simulink model "Quadrotor"  (Simulink 7.7)
settings: Solver=ode23tb  StartTime=0.0  StopTime=140  MaxStep=1e-3  RelTol=1e-3
values from neighbouring files (symbols this model uses):
  b = 54.2e-6    (= 5.42e-05)    [ParamQuadrotor.m]
  d = 1.1e-6    (= 1.1e-06)    [ParamQuadrotor.m]
  g = 9.81    [ParamQuadrotor.m]
  h = 1e-3    (= 0.001)    [ParamQuadrotor.m]
  Ixx = 8.1e-3    (= 0.0081)    [ParamQuadrotor.m]
  Iyy = 8.1e-3    (= 0.0081)    [ParamQuadrotor.m]
  Izz = 14.2e-3    (= 0.0142)    [ParamQuadrotor.m]
  Jtp = 104e-6    (= 0.000104)    [ParamQuadrotor.m]
  Kd_angle = 10*2    (= 20)    [ParamQuadrotor.m]
  Kd_motor = 0    [ParamQuadrotor.m]
  Kd_position = 10    [ParamQuadrotor.m]
  Ke = 6.3e-3    (= 0.0063)    [ParamQuadrotor.m]
  Ki_angle = 0    [ParamQuadrotor.m]
  Ki_motor = 10    [ParamQuadrotor.m]
  Ki_position = 0    [ParamQuadrotor.m]
  Km = 6.3e-3    (= 0.0063)    [ParamQuadrotor.m]
  Kp_angle = 5*2    (= 10)    [ParamQuadrotor.m]
  Kp_motor = 1    [ParamQuadrotor.m]
  Kp_position = 5    [ParamQuadrotor.m]
  l = 0.24    [ParamQuadrotor.m]
  m = 1    [ParamQuadrotor.m]
  n = 0.9    [ParamQuadrotor.m]
  N = 5.6    [ParamQuadrotor.m]
  R = 0.6    [ParamQuadrotor.m]
undefined symbols (not defined in the file or in its folder): Newton, Raphson
libraries: simulink x10
settings Model: Creator=hts  LastModifiedBy=Tai-Sik
settings SFSimCC: SimParseCustomCode=off

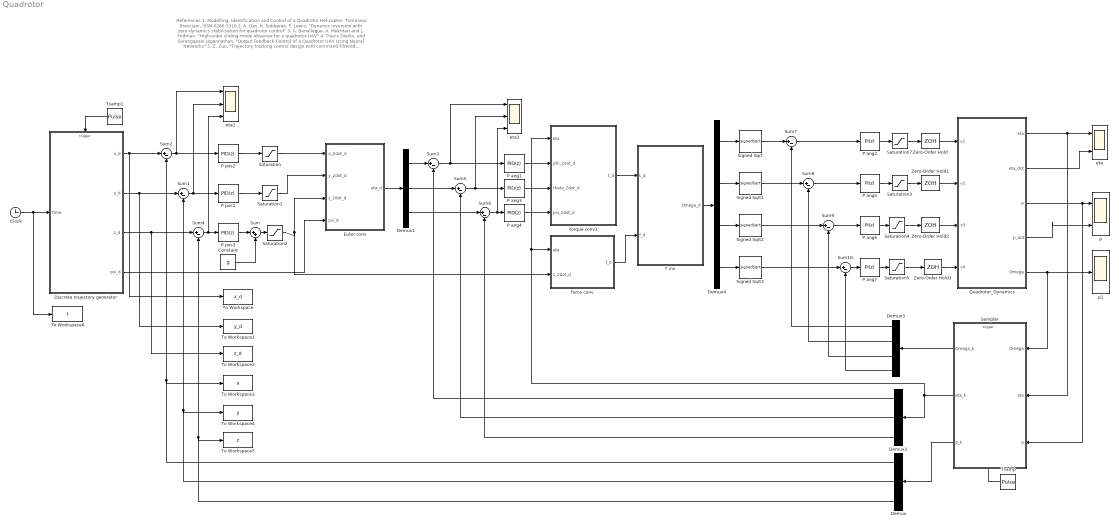
== system Quadrotor ==
  note: References
      | 1. Modelling, Identification and Control
      | of a Quadrotor Helicopter, Tommaso Bresciani, ISSN 0280-5316
      | 2. A. Das, K. Subbarao, F. Lewis, "Dynamic inversion with zero-dynamics
      | stabilisation for quadrotor control"
      | 3. A. Benallegue, A. Mokhtari and L. Fridman, "High-order sliding-mode observer for a quadrotor UAV"
      | 4. Travis Dierks, and Sarangapani Jagannathan, "Output Feedback Control of a Quadrotor UAV Using Neural Networks"
      | 5. Z. Zuo, "Trajectory tracking control design with command-filtered compensation for a quadrotor"
  Clock : Clock
      settings: Decimation=10
  Constant : Constant  Value=g
  Demux : Demux  Outputs=3
  Demux1 : Demux  Outputs=3
  Demux2 : Demux  Outputs=3
  Demux3 : Demux
  Demux4 : Demux
  Discrete trajectory generator : Subsystem  TreatAsAtomicUnit=on
  Euler conv : Stateflow chart  TreatAsAtomicUnit=on
  P ang1 : simulink/Continuous/PID Controller  SystemSampleTime=-1  Controller=PID  TimeDomain=Discrete-time  SampleTime=h  IntegratorMethod=Trapezoidal  FilterMethod=Trapezoidal  Form=Parallel  P=Kp_angle  I=Ki_angle  D=Kd_angle  N=100  InitialConditionSource=internal  InitialConditionForIntegrator=0  InitialConditionForFilter=0  ExternalReset=none  LimitOutput=off  UpperSaturationLimit=inf  LowerSaturationLimit=-inf  LinearizeAsGain=off  AntiWindupMode=none  Kb=1  TrackingMode=off  Kt=1  PParamMin=[]  PParamMax=[]  IParamMin=[]  IParamMax=[]  DParamMin=[]  DParamMax=[]  NParamMin=[]  NParamMax=[]  KbParamMin=[]  KbParamMax=[]  KtParamMin=[]  KtParamMax=[]  POutMin=[]  POutMax=[]  IOutMin=[]  IOutMax=[]  DOutMin=[]  DOutMax=[]  NOutMin=[]  NOutMax=[]  KbOutMin=[]  KbOutMax=[]  KtOutMin=[]  KtOutMax=[]  IntegratorOutMin=[]  IntegratorOutMax=[]  FilterOutMin=[]  FilterOutMax=[]  SumOutMin=[]  SumOutMax=[]  SumI1OutMin=[]  SumI1OutMax=[]  SumI2OutMin=[]  SumI2OutMax=[]  SumI3OutMin=[]  SumI3OutMax=[]  SumDOutMin=[]  SumDOutMax=[]  SaturationOutMin=[]  SaturationOutMax=[]  IntegratorContinuousStateAttributes=''  IntegratorStateMustResolveToSignalObject=off  IntegratorRTWStateStorageClass=Auto  FilterContinuousStateAttributes=''  FilterStateMustResolveToSignalObject=off  FilterRTWStateStorageClass=Auto
  P ang{2,5..7} (4 alike) : simulink/Continuous/PID Controller  SystemSampleTime=-1  Controller=PI  TimeDomain=Discrete-time  SampleTime=h  IntegratorMethod=Trapezoidal  FilterMethod=Trapezoidal  Form=Parallel  P=Kp_motor  I=Ki_motor  D=Kd_motor  N=100  InitialConditionSource=internal  InitialConditionForIntegrator=0  InitialConditionForFilter=0  ExternalReset=none  LimitOutput=off  UpperSaturationLimit=inf  LowerSaturationLimit=-inf  LinearizeAsGain=off  AntiWindupMode=none  Kb=1  TrackingMode=off  Kt=1  PParamMin=[]  PParamMax=[]  IParamMin=[]  IParamMax=[]  DParamMin=[]  DParamMax=[]  NParamMin=[]  NParamMax=[]  KbParamMin=[]  KbParamMax=[]  KtParamMin=[]  KtParamMax=[]  POutMin=[]  POutMax=[]  IOutMin=[]  IOutMax=[]  DOutMin=[]  DOutMax=[]  NOutMin=[]  NOutMax=[]  KbOutMin=[]  KbOutMax=[]  KtOutMin=[]  KtOutMax=[]  IntegratorOutMin=[]  IntegratorOutMax=[]  FilterOutMin=[]  FilterOutMax=[]  SumOutMin=[]  SumOutMax=[]  SumI1OutMin=[]  SumI1OutMax=[]  SumI2OutMin=[]  SumI2OutMax=[]  SumI3OutMin=[]  SumI3OutMax=[]  SumDOutMin=[]  SumDOutMax=[]  SaturationOutMin=[]  SaturationOutMax=[]  IntegratorContinuousStateAttributes=''  IntegratorStateMustResolveToSignalObject=off  IntegratorRTWStateStorageClass=Auto  FilterContinuousStateAttributes=''  FilterStateMustResolveToSignalObject=off  FilterRTWStateStorageClass=Auto
  P ang3 : simulink/Continuous/PID Controller  SystemSampleTime=-1  Controller=PID  TimeDomain=Discrete-time  SampleTime=h  IntegratorMethod=Trapezoidal  FilterMethod=Trapezoidal  Form=Parallel  P=Kp_angle  I=Ki_angle  D=Kd_angle  N=100  InitialConditionSource=internal  InitialConditionForIntegrator=0  InitialConditionForFilter=0  ExternalReset=none  LimitOutput=off  UpperSaturationLimit=inf  LowerSaturationLimit=-inf  LinearizeAsGain=off  AntiWindupMode=none  Kb=1  TrackingMode=off  Kt=1  PParamMin=[]  PParamMax=[]  IParamMin=[]  IParamMax=[]  DParamMin=[]  DParamMax=[]  NParamMin=[]  NParamMax=[]  KbParamMin=[]  KbParamMax=[]  KtParamMin=[]  KtParamMax=[]  POutMin=[]  POutMax=[]  IOutMin=[]  IOutMax=[]  DOutMin=[]  DOutMax=[]  NOutMin=[]  NOutMax=[]  KbOutMin=[]  KbOutMax=[]  KtOutMin=[]  KtOutMax=[]  IntegratorOutMin=[]  IntegratorOutMax=[]  FilterOutMin=[]  FilterOutMax=[]  SumOutMin=[]  SumOutMax=[]  SumI1OutMin=[]  SumI1OutMax=[]  SumI2OutMin=[]  SumI2OutMax=[]  SumI3OutMin=[]  SumI3OutMax=[]  SumDOutMin=[]  SumDOutMax=[]  SaturationOutMin=[]  SaturationOutMax=[]  IntegratorContinuousStateAttributes=''  IntegratorStateMustResolveToSignalObject=off  IntegratorRTWStateStorageClass=Auto  FilterContinuousStateAttributes=''  FilterStateMustResolveToSignalObject=off  FilterRTWStateStorageClass=Auto
  P ang4 : simulink/Continuous/PID Controller  SystemSampleTime=-1  Controller=PID  TimeDomain=Discrete-time  SampleTime=h  IntegratorMethod=Trapezoidal  FilterMethod=Trapezoidal  Form=Parallel  P=Kp_angle  I=Ki_angle  D=Kd_angle  N=100  InitialConditionSource=internal  InitialConditionForIntegrator=0  InitialConditionForFilter=0  ExternalReset=none  LimitOutput=off  UpperSaturationLimit=inf  LowerSaturationLimit=-inf  LinearizeAsGain=off  AntiWindupMode=none  Kb=1  TrackingMode=off  Kt=1  PParamMin=[]  PParamMax=[]  IParamMin=[]  IParamMax=[]  DParamMin=[]  DParamMax=[]  NParamMin=[]  NParamMax=[]  KbParamMin=[]  KbParamMax=[]  KtParamMin=[]  KtParamMax=[]  POutMin=[]  POutMax=[]  IOutMin=[]  IOutMax=[]  DOutMin=[]  DOutMax=[]  NOutMin=[]  NOutMax=[]  KbOutMin=[]  KbOutMax=[]  KtOutMin=[]  KtOutMax=[]  IntegratorOutMin=[]  IntegratorOutMax=[]  FilterOutMin=[]  FilterOutMax=[]  SumOutMin=[]  SumOutMax=[]  SumI1OutMin=[]  SumI1OutMax=[]  SumI2OutMin=[]  SumI2OutMax=[]  SumI3OutMin=[]  SumI3OutMax=[]  SumDOutMin=[]  SumDOutMax=[]  SaturationOutMin=[]  SaturationOutMax=[]  IntegratorContinuousStateAttributes=''  IntegratorStateMustResolveToSignalObject=off  IntegratorRTWStateStorageClass=Auto  FilterContinuousStateAttributes=''  FilterStateMustResolveToSignalObject=off  FilterRTWStateStorageClass=Auto
  P pos1 : simulink/Continuous/PID Controller  SystemSampleTime=-1  Controller=PID  TimeDomain=Discrete-time  SampleTime=h  IntegratorMethod=Trapezoidal  FilterMethod=Trapezoidal  Form=Parallel  P=Kp_position  I=Ki_position  D=Kd_position  N=100  InitialConditionSource=internal  InitialConditionForIntegrator=0  InitialConditionForFilter=0  ExternalReset=none  LimitOutput=off  UpperSaturationLimit=5  LowerSaturationLimit=-10  LinearizeAsGain=off  AntiWindupMode=none  Kb=1  TrackingMode=off  Kt=1  PParamMin=[]  PParamMax=[]  IParamMin=[]  IParamMax=[]  DParamMin=[]  DParamMax=[]  NParamMin=[]  NParamMax=[]  KbParamMin=[]  KbParamMax=[]  KtParamMin=[]  KtParamMax=[]  POutMin=[]  POutMax=[]  IOutMin=[]  IOutMax=[]  DOutMin=[]  DOutMax=[]  NOutMin=[]  NOutMax=[]  KbOutMin=[]  KbOutMax=[]  KtOutMin=[]  KtOutMax=[]  IntegratorOutMin=[]  IntegratorOutMax=[]  FilterOutMin=[]  FilterOutMax=[]  SumOutMin=[]  SumOutMax=[]  SumI1OutMin=[]  SumI1OutMax=[]  SumI2OutMin=[]  SumI2OutMax=[]  SumI3OutMin=[]  SumI3OutMax=[]  SumDOutMin=[]  SumDOutMax=[]  SaturationOutMin=[]  SaturationOutMax=[]  IntegratorContinuousStateAttributes=''  IntegratorStateMustResolveToSignalObject=off  IntegratorRTWStateStorageClass=Auto  FilterContinuousStateAttributes=''  FilterStateMustResolveToSignalObject=off  FilterRTWStateStorageClass=Auto
  P pos2 : simulink/Continuous/PID Controller  SystemSampleTime=-1  Controller=PID  TimeDomain=Discrete-time  SampleTime=h  IntegratorMethod=Trapezoidal  FilterMethod=Trapezoidal  Form=Parallel  P=Kp_position  I=Ki_position  D=Kd_position  N=100  InitialConditionSource=internal  InitialConditionForIntegrator=0  InitialConditionForFilter=0  ExternalReset=none  LimitOutput=off  UpperSaturationLimit=5  LowerSaturationLimit=-10  LinearizeAsGain=off  AntiWindupMode=none  Kb=1  TrackingMode=off  Kt=1  PParamMin=[]  PParamMax=[]  IParamMin=[]  IParamMax=[]  DParamMin=[]  DParamMax=[]  NParamMin=[]  NParamMax=[]  KbParamMin=[]  KbParamMax=[]  KtParamMin=[]  KtParamMax=[]  POutMin=[]  POutMax=[]  IOutMin=[]  IOutMax=[]  DOutMin=[]  DOutMax=[]  NOutMin=[]  NOutMax=[]  KbOutMin=[]  KbOutMax=[]  KtOutMin=[]  KtOutMax=[]  IntegratorOutMin=[]  IntegratorOutMax=[]  FilterOutMin=[]  FilterOutMax=[]  SumOutMin=[]  SumOutMax=[]  SumI1OutMin=[]  SumI1OutMax=[]  SumI2OutMin=[]  SumI2OutMax=[]  SumI3OutMin=[]  SumI3OutMax=[]  SumDOutMin=[]  SumDOutMax=[]  SaturationOutMin=[]  SaturationOutMax=[]  IntegratorContinuousStateAttributes=''  IntegratorStateMustResolveToSignalObject=off  IntegratorRTWStateStorageClass=Auto  FilterContinuousStateAttributes=''  FilterStateMustResolveToSignalObject=off  FilterRTWStateStorageClass=Auto
  P pos3 : simulink/Continuous/PID Controller  SystemSampleTime=-1  Controller=PID  TimeDomain=Discrete-time  SampleTime=h  IntegratorMethod=Trapezoidal  FilterMethod=Trapezoidal  Form=Parallel  P=Kp_position  I=Ki_position  D=Kd_position  N=100  InitialConditionSource=internal  InitialConditionForIntegrator=0  InitialConditionForFilter=0  ExternalReset=none  LimitOutput=off  UpperSaturationLimit=5  LowerSaturationLimit=-10  LinearizeAsGain=off  AntiWindupMode=none  Kb=1  TrackingMode=off  Kt=1  PParamMin=[]  PParamMax=[]  IParamMin=[]  IParamMax=[]  DParamMin=[]  DParamMax=[]  NParamMin=[]  NParamMax=[]  KbParamMin=[]  KbParamMax=[]  KtParamMin=[]  KtParamMax=[]  POutMin=[]  POutMax=[]  IOutMin=[]  IOutMax=[]  DOutMin=[]  DOutMax=[]  NOutMin=[]  NOutMax=[]  KbOutMin=[]  KbOutMax=[]  KtOutMin=[]  KtOutMax=[]  IntegratorOutMin=[]  IntegratorOutMax=[]  FilterOutMin=[]  FilterOutMax=[]  SumOutMin=[]  SumOutMax=[]  SumI1OutMin=[]  SumI1OutMax=[]  SumI2OutMin=[]  SumI2OutMax=[]  SumI3OutMin=[]  SumI3OutMax=[]  SumDOutMin=[]  SumDOutMax=[]  SaturationOutMin=[]  SaturationOutMax=[]  IntegratorContinuousStateAttributes=''  IntegratorStateMustResolveToSignalObject=off  IntegratorRTWStateStorageClass=Auto  FilterContinuousStateAttributes=''  FilterStateMustResolveToSignalObject=off  FilterRTWStateStorageClass=Auto
  Quadrotor_Dynamics : Subsystem
  Sampler : Subsystem  TreatAsAtomicUnit=on
  Saturation : Saturate  UpperLimit=3*g  LowerLimit=-3*g
  Saturation1 : Saturate  UpperLimit=3*g  LowerLimit=-3*g
  Saturation2 : Saturate  UpperLimit=3*g  LowerLimit=-3*g
  Saturation{3..5,7} (4 alike) : Saturate  UpperLimit=100  LowerLimit=-100
  Signed Sqrt{,1..3} (4 alike) : Sqrt  Operator=signedSqrt  AlgorithmType=Newton-Raphson  SaturateOnIntegerOverflow=on
  Sum : Sum  Inputs=|++
  Sum{1..10} (10 alike) : Sum  Inputs=|+-
  T inv : Stateflow chart  TreatAsAtomicUnit=on
  To Workspace : ToWorkspace  VariableName=x_d  SampleTime=h*10  SaveFormat=Array
  To Workspace1 : ToWorkspace  VariableName=y_d  SampleTime=h*10  SaveFormat=Array
  To Workspace2 : ToWorkspace  VariableName=z_d  SampleTime=h*10  SaveFormat=Array
  To Workspace3 : ToWorkspace  VariableName=x  SampleTime=h*10  SaveFormat=Array
  To Workspace4 : ToWorkspace  VariableName=y  SampleTime=h*10  SaveFormat=Array
  To Workspace5 : ToWorkspace  VariableName=z  SampleTime=h*10  SaveFormat=Array
  To Workspace6 : ToWorkspace  VariableName=t  SampleTime=h*10  SaveFormat=Array
  Tsamp : DiscretePulseGenerator  PulseType=Time based  Period=h  PulseWidth=50
  Tsamp1 : DiscretePulseGenerator  PulseType=Time based  Period=h  PulseWidth=50
  Zero-Order Hold{,1..3} (4 alike) : ZeroOrderHold  SampleTime=h
  eta : Scope  NumInputPorts=2
      settings: TimeRange=20  YMin=-0.1~-1.75  YMax=0.55~1
  eta1 : Scope  NumInputPorts=3
      settings: TimeRange=20  YMin=-0.4~0.05~0.14  YMax=0.4~0.4~0.18  SaveName=ScopeData5
  eta2 : Scope  NumInputPorts=3
      settings: TimeRange=20  YMin=-0.275~-0.275~-0.03  YMax=0.1~0.1~0.06  SaveName=ScopeData6
  force conv : Stateflow chart  TreatAsAtomicUnit=on
  p : Scope  NumInputPorts=2
      settings: TimeRange=80  YMin=0~0  YMax=20~2.75
  p1 : Scope
      settings: TimeRange=0.7000000000000001  YMin=213.268  YMax=213.31  SaveName=ScopeData4
  torque conv1 : Stateflow chart  TreatAsAtomicUnit=on
  wires:
  Quadrotor_Dynamics/1(eta) -> eta/1, Sampler/2(eta)
  Quadrotor_Dynamics/3(p) -> p/1, Sampler/3(p)
  Sum4/1 -> P pos3/1, eta1/3
  Discrete trajectory generator/3(z_d) -> Sum4/1, To Workspace2/1
  P pos3/1 -> Sum/1
  Sum/1 -> Saturation2/1
  Sum1/1 -> P pos1/1, eta1/2
  Discrete trajectory generator/2(y_d) -> Sum1/1, To Workspace1/1
  Sum2/1 -> P pos2/1, eta1/1
  Discrete trajectory generator/1(x_d) -> Sum2/1, To Workspace/1
  P pos2/1 -> Saturation/1
  P pos1/1 -> Saturation1/1
  Sum3/1 -> P ang1/1, eta2/1
  Sum5/1 -> P ang3/1, eta2/2
  Sum6/1 -> P ang4/1, eta2/3
  Demux2/1 -> Sum3/2
  Demux2/2 -> Sum5/2
  Demux2/3 -> Sum6/2
  P ang1/1 -> torque conv1/2(phi_2dot_d)
  P ang3/1 -> torque conv1/3(theta_2dot_d)
  P ang4/1 -> torque conv1/4(psi_2dot_d)
  Saturation2/1 -> force conv/2(z_2dot_d), Euler conv/3(z_2dot_d)
  Constant/1 -> Sum/2
  Demux1/1 -> Sum3/1
  Demux1/2 -> Sum5/1
  Saturation/1 -> Euler conv/1(x_2dot_d)
  Saturation1/1 -> Euler conv/2(y_2dot_d)
  Euler conv/1(eta_d) -> Demux1/1
  Demux1/3 -> Sum6/1
  Demux/1 -> Sum2/2, To Workspace3/1
  Demux/2 -> Sum1/2, To Workspace4/1
  Demux/3 -> Sum4/2, To Workspace5/1
  Tsamp/1 -> Sampler/Trigger
  Sampler/1(Omega_k) -> Demux3/1
  Sampler/3(p_k) -> Demux/1
  Quadrotor_Dynamics/5(Omega) -> Sampler/1(Omega), p1/1
  torque conv1/1(t_d) -> T inv/1(t_d)
  force conv/1(f_d) -> T inv/2(f_d)
  Sampler/2(eta_k) -> Demux2/1, force conv/1(eta), torque conv1/1(eta)
  Demux4/1 -> Signed Sqrt/1
  Sum7/1 -> P ang2/1
  Demux3/1 -> Sum7/2
  Demux4/2 -> Signed Sqrt1/1
  Demux4/4 -> Signed Sqrt3/1
  Sum8/1 -> P ang5/1
  Demux3/2 -> Sum8/2
  Demux3/3 -> Sum9/2
  Sum9/1 -> P ang6/1
  Sum10/1 -> P ang7/1
  Demux3/4 -> Sum10/2
  P ang2/1 -> Saturation7/1
  P ang5/1 -> Saturation3/1
  P ang6/1 -> Saturation4/1
  P ang7/1 -> Saturation5/1
  Demux4/3 -> Signed Sqrt2/1
  Zero-Order Hold/1 -> Quadrotor_Dynamics/1(v1)
  Zero-Order Hold1/1 -> Quadrotor_Dynamics/2(v2)
  Zero-Order Hold2/1 -> Quadrotor_Dynamics/3(v3)
  Zero-Order Hold3/1 -> Quadrotor_Dynamics/4(v4)
  Saturation7/1 -> Zero-Order Hold/1
  Saturation3/1 -> Zero-Order Hold1/1
  Saturation4/1 -> Zero-Order Hold2/1
  Saturation5/1 -> Zero-Order Hold3/1
  T inv/1(Omega_d) -> Demux4/1
  Signed Sqrt/1 -> Sum7/1
  Signed Sqrt1/1 -> Sum8/1
  Signed Sqrt2/1 -> Sum9/1
  Signed Sqrt3/1 -> Sum10/1
  Discrete trajectory generator/4(psi_d) -> Euler conv/4(psi_d)
  Tsamp1/1 -> Discrete trajectory generator/Trigger
  Clock/1 -> Discrete trajectory generator/1(Time), To Workspace6/1
  Quadrotor_Dynamics/2(eta_dot) -> eta/2
  Quadrotor_Dynamics/4(p_dot) -> p/2

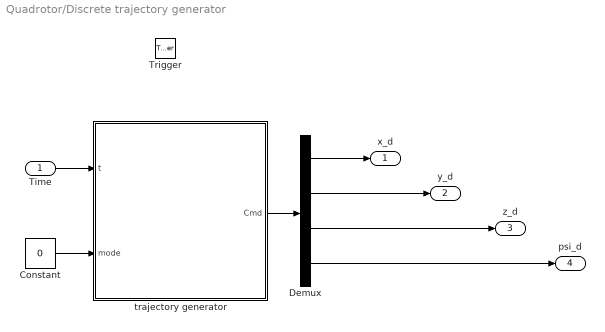
== system Quadrotor/Discrete trajectory generator ==
  Time : Inport
  Trigger : TriggerPort
  Constant : Constant  Value=0
  Demux : Demux
  trajectory generator : Stateflow chart  TreatAsAtomicUnit=on
  x_d : Outport
  y_d : Outport  Port=2
  z_d : Outport  Port=3
  psi_d : Outport  Port=4
  wires:
  Time/1 -> trajectory generator/1(t)
  trajectory generator/1(Cmd) -> Demux/1
  Demux/1 -> x_d/1
  Demux/2 -> y_d/1
  Demux/3 -> z_d/1
  Demux/4 -> psi_d/1
  Constant/1 -> trajectory generator/2(mode)

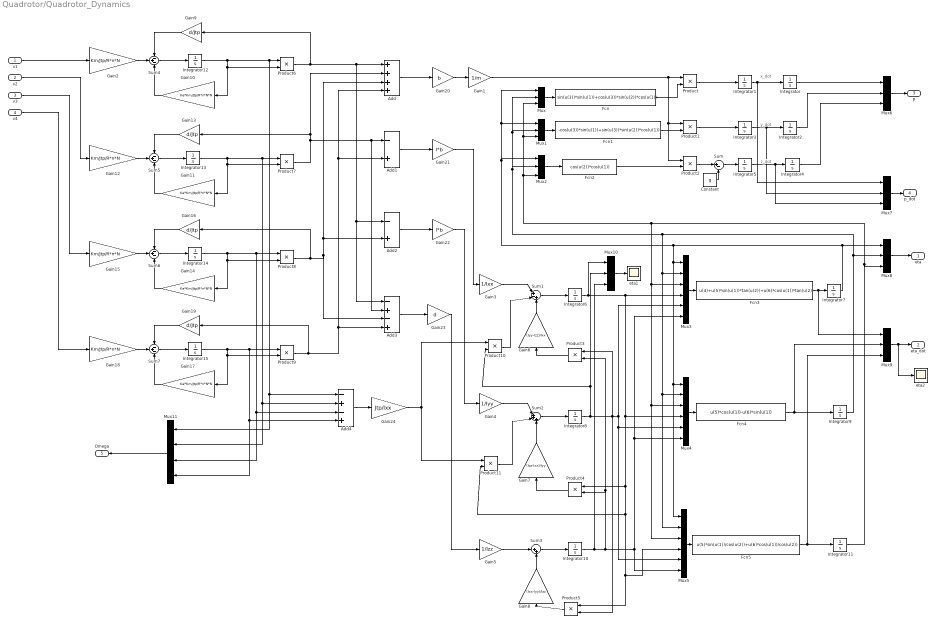
== system Quadrotor/Quadrotor_Dynamics ==
  note: x_dot
  note: y_dot
  note: z_dot
  v1 : Inport
  v2 : Inport  Port=2
  v3 : Inport  Port=3
  v4 : Inport  Port=4
  Add : Sum  Inputs=++++
  Add1 : Sum  Inputs=-+
  Add2 : Sum  Inputs=-+
  Add3 : Sum  Inputs=-+-+
  Add4 : Sum  Inputs=-+-+
  Constant : Constant  Value=g
  Fcn : Fcn  Expr=sin(u(3))*sin(u(1))+cos(u(3))*sin(u(2))*cos(u(1))
  Fcn1 : Fcn  Expr=-cos(u(3))*sin(u(1))+sin(u(3))*sin(u(2))*cos(u(1))
  Fcn2 : Fcn  Expr=cos(u(2))*cos(u(1))
  Fcn3 : Fcn  Expr=u(4)+u(5)*sin(u(1))*tan(u(2))+u(6)*cos(u(1))*tan(u(2))
  Fcn4 : Fcn  Expr=u(5)*cos(u(1))-u(6)*sin(u(1))
  Fcn5 : Fcn  Expr=u(5)*sin(u(1))/cos(u(2))+u(6)*cos(u(1))/cos(u(2))
  Gain1 : Gain  Gain=1/m
  Gain{10..11,14,17} (4 alike) : Gain  Gain=Ke*Km/Jtp/R*n*N*N
  Gain{2,12,15,18} (4 alike) : Gain  Gain=Km/Jtp/R*n*N
  Gain{9,13,16,19} (4 alike) : Gain  Gain=d/Jtp
  Gain20 : Gain  Gain=b
  Gain21 : Gain  Gain=l*b
  Gain22 : Gain  Gain=l*b
  Gain23 : Gain  Gain=d
  Gain24 : Gain  Gain=Jtp/Ixx
  Gain3 : Gain  Gain=1/Ixx
  Gain4 : Gain  Gain=1/Iyy
  Gain5 : Gain  Gain=1/Izz
  Gain6 : Gain  Gain=(Iyy-Izz)/Ixx
  Gain7 : Gain  Gain=(Izz-Ixx)/Iyy
  Gain8 : Gain  Gain=(Ixx-Iyy)/Izz
  Integrator{,1..15} (16 alike) : Integrator
  Mux{,1..2,6..10} (8 alike) : Mux  Inputs=3
  Mux11 : Mux
  Mux3 : Mux  Inputs=6
  Mux4 : Mux  Inputs=6
  Mux5 : Mux  Inputs=6
  Product{,1..11} (12 alike) : Product  RndMeth=Zero
  Sum : Sum  Inputs=|+-
  Sum1 : Sum  Inputs=|+-+
  Sum2 : Sum  Inputs=|+++
  Sum3 : Sum  Inputs=|++
  Sum{4..7} (4 alike) : Sum  Inputs=-+-
  eta1 : Scope
      settings: TimeRange=10  YMin=-0.00225  YMax=0.003  SaveName=ScopeData2
  eta2 : Scope
      settings: TimeRange=10  YMin=-0.0008  YMax=0.0008  SaveName=ScopeData3
  eta : Outport
  eta_dot : Outport  Port=2
  p : Outport  Port=3
  p_dot : Outport  Port=4
  Omega : Outport  Port=5
  wires:
  Integrator1/1 -> Integrator/1, Mux7/1
  Product/1 -> Integrator1/1
  Mux/1 -> Fcn/1
  Fcn/1 -> Product/2
  Integrator3/1 -> Integrator2/1, Mux7/2
  Product1/1 -> Integrator3/1
  Integrator5/1 -> Integrator4/1, Mux7/3
  Mux2/1 -> Fcn2/1
  Fcn2/1 -> Product2/2
  Product2/1 -> Sum/1
  Sum/1 -> Integrator5/1
  Constant/1 -> Sum/2
  Sum1/1 -> Integrator6/1
  Fcn3/1 -> Integrator7/1, Mux9/1
  Integrator7/1 -> Mux8/1, Mux3/1, Mux4/1, Mux5/1, Mux2/1, Mux1/1, Mux/1
  Mux3/1 -> Fcn3/1
  Integrator6/1 -> Mux3/4, Product4/1, Product5/1, Mux5/4, Product11/2, Mux4/4, Mux10/1
  Sum2/1 -> Integrator8/1
  Fcn4/1 -> Integrator9/1, Mux9/2
  Integrator9/1 -> Mux8/2, Mux3/2, Mux4/2, Mux5/2, Mux/2, Mux1/2, Mux2/2
  Mux4/1 -> Fcn4/1
  Integrator8/1 -> Product5/2, Product3/1, Mux3/5, Mux4/5, Mux5/5, Mux10/2, Product10/2
  Sum3/1 -> Integrator10/1
  Gain5/1 -> Sum3/1
  Fcn5/1 -> Integrator11/1, Mux9/3
  Integrator11/1 -> Mux8/3, Mux3/3, Mux4/3, Mux5/3, Mux/3, Mux1/3, Mux2/3
  Mux5/1 -> Fcn5/1
  Integrator10/1 -> Product3/2, Product4/2, Mux3/6, Mux4/6, Mux5/6, Mux10/3
  Product3/1 -> Gain6/1
  Product4/1 -> Gain7/1
  Product5/1 -> Gain8/1
  Gain8/1 -> Sum3/2
  Mux6/1 -> p/1
  Mux7/1 -> p_dot/1
  Mux8/1 -> eta/1
  Mux9/1 -> eta_dot/1, eta2/1
  Mux10/1 -> eta1/1
  Gain1/1 -> Product/1, Product2/1, Product1/1
  Gain2/1 -> Sum4/2
  Gain9/1 -> Sum4/1
  Gain10/1 -> Sum4/3
  Integrator12/1 -> Gain10/1, Product6/2, Product6/1, Add4/1, Mux11/1
  Product6/1 -> Gain9/1, Add/1, Add2/1, Add3/1
  Gain12/1 -> Sum5/2
  Gain13/1 -> Sum5/1
  Integrator13/1 -> Gain11/1, Product7/2, Product7/1, Add4/2, Mux11/2
  Product7/1 -> Gain13/1, Add/2, Add1/1, Add3/2
  Gain15/1 -> Sum6/2
  Gain16/1 -> Sum6/1
  Gain14/1 -> Sum6/3
  Integrator14/1 -> Gain14/1, Product8/2, Product8/1, Add4/3, Mux11/3
  Product8/1 -> Gain16/1, Add/3, Add2/2, Add3/3
  Gain18/1 -> Sum7/2
  Gain19/1 -> Sum7/1
  Gain17/1 -> Sum7/3
  Integrator15/1 -> Gain17/1, Product9/2, Product9/1, Add4/4, Mux11/4
  Product9/1 -> Gain19/1, Add/4, Add1/2, Add3/4
  Mux11/1 -> Omega/1
  Gain6/1 -> Sum1/3
  Gain3/1 -> Sum1/1
  Gain7/1 -> Sum2/3
  Gain4/1 -> Sum2/1
  Product10/1 -> Sum1/2
  Product11/1 -> Sum2/2
  v1/1 -> Gain2/1
  v2/1 -> Gain12/1
  v3/1 -> Gain15/1
  v4/1 -> Gain18/1
  Gain11/1 -> Sum5/3
  Gain20/1 -> Gain1/1
  Gain21/1 -> Gain3/1
  Gain22/1 -> Gain4/1
  Gain23/1 -> Gain5/1
  Sum6/1 -> Integrator14/1
  Sum7/1 -> Integrator15/1
  Sum4/1 -> Integrator12/1
  Sum5/1 -> Integrator13/1
  Add4/1 -> Gain24/1
  Add/1 -> Gain20/1
  Add1/1 -> Gain21/1
  Add2/1 -> Gain22/1
  Add3/1 -> Gain23/1
  Mux1/1 -> Fcn1/1
  Fcn1/1 -> Product1/2
  Integrator/1 -> Mux6/1
  Integrator2/1 -> Mux6/2
  Integrator4/1 -> Mux6/3
  Gain24/1 -> Product10/1, Product11/1

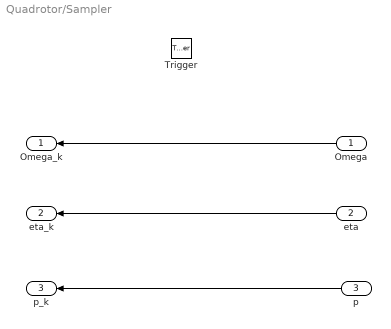
== system Quadrotor/Sampler ==
  Omega : Inport
  eta : Inport  Port=2
  p : Inport  Port=3
  Trigger : TriggerPort
  Omega_k : Outport
  eta_k : Outport  Port=2
  p_k : Outport  Port=3
  wires:
  Omega/1 -> Omega_k/1
  eta/1 -> eta_k/1
  p/1 -> p_k/1

== matlab function torque conv1 ==
  data: eta input double size=3; phi_2dot_d input double size=1; theta_2dot_d input double size=1; psi_2dot_d input double size=1; t_d output double size=3; I parameter double
function t_d = C(eta,phi_2dot_d,theta_2dot_d,psi_2dot_d,I)

tr_d = [phi_2dot_d;theta_2dot_d;psi_2dot_d];
sphi = sin(eta(1));
cphi = cos(eta(1));
stht = sin(eta(2));
ctht = cos(eta(2));
spsi = sin(eta(3));
cpsi = cos(eta(3));

C = [1   0     -stht;
     0   cphi  sphi*ctht;
     0   -sphi cphi*ctht];

%C = [1   0     0;
%     0   1     0;
%     0   0    1];

t_d = I*C*tr_d;

== matlab function T inv ==
  data: t_d input double size=3; Omega_d output double size=4; f_d input double size=1; b parameter double; l parameter double; d parameter double
function Omega_d = Inv_T(t_d, f_d, b, l, d)

T = [b    b     b     b;
     0   -l*b   0  l*b;
    -l*b   0    l*b   0;
     -d    d    -d    d];

u = [f_d; t_d(1); t_d(2); t_d(3)]; 
 
Omega_d = inv(T)*u;

== matlab function Discrete trajectory generator/trajectory generator ==
  data: t input double size=1; mode input double size=1; Cmd output double size=4
function Cmd = G(t,mode)
if mode == 1
    if t < 20
        x_d = 0;
        y_d = 0;
        z_d = 20;
    elseif t >= 20 && t < 60
        x_d = 20;
        y_d = 0;
        z_d = 20;
    elseif t >= 60 && t < 100
        x_d = 20;
        y_d = 20;
        z_d = 20;
    else
        x_d = 0;
        y_d = 20;
        z_d = 20;     
    end
else
    if t < 20
        x_d = 0;
        y_d = 0;
        z_d = 10;
    elseif t >= 20 && t < 80
        x_d = (t-20)/5*sin(2*pi*t/20);
        y_d = (t-20)/5*cos(2*pi*t/20);
        z_d = 20;
    else
        x_d = 12*sin(2*pi*t/20);
        y_d = 12*cos(2*pi*t/20);
        z_d = 20;     
    end
end    
psi_d = pi/6;
Cmd = [x_d;y_d;z_d;psi_d];

== matlab function force conv ==
  data: eta input double size=3; z_2dot_d input double size=1; f_d output double; m parameter double
function f_d = R(eta, z_2dot_d, m)

sphi = sin(eta(1));
cphi = cos(eta(1));
stht = sin(eta(2));
ctht = cos(eta(2));
spsi = sin(eta(3));
cpsi = cos(eta(3));

R = [cpsi*ctht cpsi*stht*sphi-spsi*cphi cpsi*stht*cphi+spsi*sphi;	
     spsi*ctht spsi*stht*sphi+cpsi*cphi spsi*stht*cphi-cpsi*sphi;	
     -stht     ctht*sphi                ctht*cphi];

u = [0; 0; z_2dot_d];
d = m*inv(R)*u;

f_d = d(3);

== matlab function Euler conv ==
  data: x_2dot_d input double size=1; y_2dot_d input double size=1; z_2dot_d input double size=1; psi_d input double size=1; eta_d output double size=3
function eta_d = E(x_2dot_d,y_2dot_d,z_2dot_d,psi_d)

d = sqrt(x_2dot_d*x_2dot_d + y_2dot_d*y_2dot_d + z_2dot_d*z_2dot_d);

if -0.001 < d && d < 0.001
    phi_d = 0;
else
    phi_d = asin((x_2dot_d*sin(psi_d) - y_2dot_d*cos(psi_d))/d);
end

theta_d = atan2(x_2dot_d*cos(psi_d) + y_2dot_d*sin(psi_d), z_2dot_d);

min_ang = -pi/6;
max_ang =  pi/6;

if phi_d < min_ang 
    phi_d = min_ang; 
end
if phi_d > max_ang 
    phi_d = max_ang; 
end
if theta_d < min_ang 
    theta_d = min_ang; 
end
if theta_d > max_ang
    theta_d = max_ang; 
end
eta_d= [phi_d; theta_d; psi_d];
